simulink subsystem "BrakingHydraulicsDiscBrakesSSC"  (R2023a)
settings: Solver=VariableStepAuto  StartTime=0.0  StopTime=10.0  RelTol=1e-3
undefined symbols (not defined in the file): AxlFL, AxlFR, AxlRL, AxlRR, PlntBrkFrntBias, PlntBrkPrsFctr, PlntBrkRearBias
libraries: sdl_lib x4, nesl_utility_internal x4, autolibutils x1
settings Model: Creator=The MathWorks, Inc.  LastModifiedBy=The MathWorks, Inc.
settings OptimizationCC: ReuseModelBlockBuffer=off

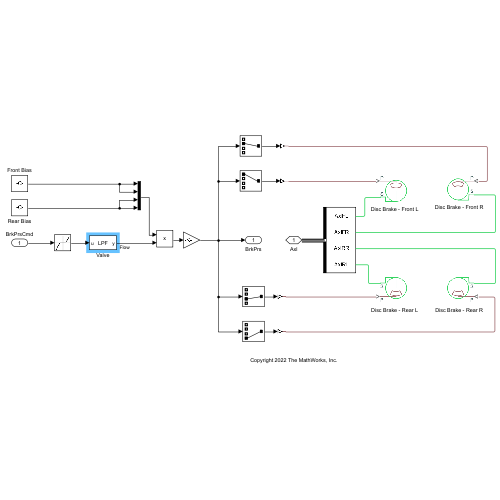
[thumbnail: Simulink's stored preview of the top-level diagram]
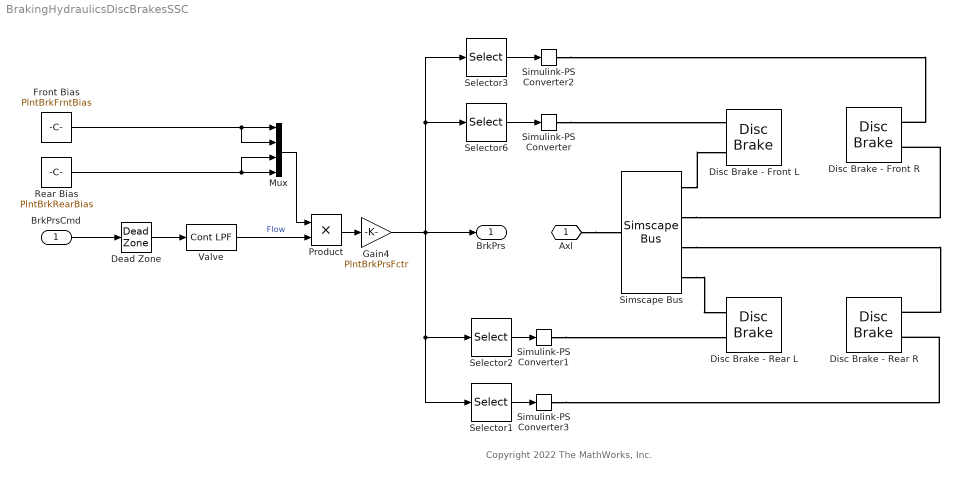
== system BrakingHydraulicsDiscBrakesSSC ==
  note: Copyright 2022 The MathWorks, Inc.
  BrkPrsCmd : Inport
  Dead Zone : DeadZone  LowerValue=-inf  UpperValue=1e-3  ZeroCross=off
  Disc Brake - Front L : sdl_lib/Brakes & Detents/Rotational/Disc Brake  r_mean=PlntBrkPadMeanRadiusFrnt m  bore=PlntBrkActrBoreFrnt m  n_pads=PlntBrkNumPadsFrnt  thermal_port=simscape.enum.thermaleffects.omit  mu_static=PlntBrkStcFricCffFrnt  mu_coulomb=PlntBrkKinFricCffFrnt  temperature_TLU=[280, 300, 320] K  mu_static_TLU=[.9, .8, .7]  mu_coulomb_TLU=[.8, .7, .6]  brkwy_vel=PlntBrkBreakFricVelFrnt rad/s  visc_coef=PlntBrkViscFricFrnt N*m*s/rad  enable_faults=simscape.enum.onoff.off  faulted_pressure=0 bar  external_fault=simscape.enum.onoff.off  temporal_fault=simscape.enum.onoff.off  fault_time=5 s  report_fault=simscape.enum.assert.action.none  thermal_mass=50 kJ/K  temperature_specify=off  temperature_priority=High  temperature=300 K  temperature_nominal_specify=off  temperature_nominal_unit=K  temperature_nominal_value=1
      settings: SourceProductName=Driveline
  Disc Brake - Front R : sdl_lib/Brakes & Detents/Rotational/Disc Brake  r_mean=PlntBrkPadMeanRadiusFrnt m  bore=PlntBrkActrBoreFrnt m  n_pads=PlntBrkNumPadsFrnt  thermal_port=simscape.enum.thermaleffects.omit  mu_static=PlntBrkStcFricCffFrnt  mu_coulomb=PlntBrkKinFricCffFrnt  temperature_TLU=[280, 300, 320] K  mu_static_TLU=[.9, .8, .7]  mu_coulomb_TLU=[.8, .7, .6]  brkwy_vel=PlntBrkBreakFricVelFrnt rad/s  visc_coef=PlntBrkViscFricFrnt N*m*s/rad  enable_faults=simscape.enum.onoff.off  faulted_pressure=0 bar  external_fault=simscape.enum.onoff.off  temporal_fault=simscape.enum.onoff.off  fault_time=5 s  report_fault=simscape.enum.assert.action.none  thermal_mass=50 kJ/K  temperature_specify=off  temperature_priority=High  temperature=300 K  temperature_nominal_specify=off  temperature_nominal_unit=K  temperature_nominal_value=1
      settings: SourceProductName=Driveline
  Disc Brake - Rear L : sdl_lib/Brakes & Detents/Rotational/Disc Brake  r_mean=PlntBrkPadMeanRadiusRear m  bore=PlntBrkActrBoreRear m  n_pads=PlntBrkNumPadsRear  thermal_port=simscape.enum.thermaleffects.omit  mu_static=PlntBrkStcFricCffRear  mu_coulomb=PlntBrkKinFricCffRear  temperature_TLU=[280, 300, 320] K  mu_static_TLU=[.9, .8, .7]  mu_coulomb_TLU=[.8, .7, .6]  brkwy_vel=PlntBrkBreakFricVelRear rad/s  visc_coef=PlntBrkViscFricRear N*m*s/rad  enable_faults=simscape.enum.onoff.off  faulted_pressure=0 bar  external_fault=simscape.enum.onoff.off  temporal_fault=simscape.enum.onoff.off  fault_time=5 s  report_fault=simscape.enum.assert.action.none  thermal_mass=50 kJ/K  temperature_specify=off  temperature_priority=High  temperature=300 K  temperature_nominal_specify=off  temperature_nominal_unit=K  temperature_nominal_value=1
      settings: SourceProductName=Driveline
  Disc Brake - Rear R : sdl_lib/Brakes & Detents/Rotational/Disc Brake  r_mean=PlntBrkPadMeanRadiusRear m  bore=PlntBrkActrBoreRear m  n_pads=PlntBrkNumPadsRear  thermal_port=simscape.enum.thermaleffects.omit  mu_static=PlntBrkStcFricCffRear  mu_coulomb=PlntBrkKinFricCffRear  temperature_TLU=[280, 300, 320] K  mu_static_TLU=[.9, .8, .7]  mu_coulomb_TLU=[.8, .7, .6]  brkwy_vel=PlntBrkBreakFricVelRear rad/s  visc_coef=PlntBrkViscFricRear N*m*s/rad  enable_faults=simscape.enum.onoff.off  faulted_pressure=0 bar  external_fault=simscape.enum.onoff.off  temporal_fault=simscape.enum.onoff.off  fault_time=5 s  report_fault=simscape.enum.assert.action.none  thermal_mass=50 kJ/K  temperature_specify=off  temperature_priority=High  temperature=300 K  temperature_nominal_specify=off  temperature_nominal_unit=K  temperature_nominal_value=1
      settings: SourceProductName=Driveline
  Front Bias : Constant  Value=PlntBrkFrntBias  SampleTime=-1
  Gain4 : Gain  Gain=PlntBrkPrsFctr
  Mux : Mux
  Product : Product
  Rear Bias : Constant  Value=PlntBrkRearBias  SampleTime=-1
  Selector1 : Selector  InputPortWidth=4  IndexOptions=Index vector (dialog)  Indices=[4]  OutputSizes=1
  Selector2 : Selector  InputPortWidth=4  IndexOptions=Index vector (dialog)  Indices=[3]  OutputSizes=1
  Selector3 : Selector  InputPortWidth=4  IndexOptions=Index vector (dialog)  Indices=[2]  OutputSizes=1
  Selector6 : Selector  InputPortWidth=4  IndexOptions=Index vector (dialog)  Indices=[1]  OutputSizes=1
  Simscape Bus : SimscapeBus  HierarchyStrings=AxlFL;AxlFR;AxlRR;AxlRL
  Simulink-PS Converter{,1..3} (4 alike) : nesl_utility_internal/Simulink-PS Converter  PhysicalDomain=network_engine_domain  SubClassName=ps_input  LeftPortType=input  RightPortType=output  PseudoPeriodic=off  Frequencies=[]  NoiseDistribution=none  NoiseParameters=[]  Unit=Pa  AffineConversion=off  FilteringAndDerivatives=provide  SimscapeFilterOrder=1  InputFilterTimeConstant=0.001  UdotUserProvided=0
  Valve : autolibutils/Cont LPF  wc=PlntBrkWc  AbsoluteTolerance=auto  aMode=6
  Axl : PMIOPort  Side=Right
  BrkPrs : Outport  VectorParamsAs1DForOutWhenUnconnected=off
  wires:
  Rear Bias/1 -> Mux/3, Mux/4
  BrkPrsCmd/1 -> Dead Zone/1
  Front Bias/1 -> Mux/2, Mux/1
  Selector1/1 -> Simulink-PS Converter3/1
  Product/1 -> Gain4/1
  Mux/1 -> Product/1
  Valve/1 -> Product/2  "Flow"
  Dead Zone/1 -> Valve/1
  Selector3/1 -> Simulink-PS Converter2/1
  Gain4/1 -> Selector3/1, Selector6/1, BrkPrs/1, Selector2/1, Selector1/1
  Selector2/1 -> Simulink-PS Converter1/1
  Selector6/1 -> Simulink-PS Converter/1
  connections:
  Simscape Bus/LConn3 -- Disc Brake - Rear R/LConn2
  Axl/RConn1 -- Simscape Bus/RConn1
  Simscape Bus/LConn1 -- Disc Brake - Front L/LConn2
  Simscape Bus/LConn4 -- Disc Brake - Rear L/LConn2
  Simulink-PS Converter3/RConn1 -- Disc Brake - Rear R/LConn1
  Simulink-PS Converter2/RConn1 -- Disc Brake - Front R/LConn1
  Simulink-PS Converter/RConn1 -- Disc Brake - Front L/LConn1
  Simscape Bus/LConn2 -- Disc Brake - Front R/LConn2
  Simulink-PS Converter1/RConn1 -- Disc Brake - Rear L/LConn1
